simulink model "sixth"  (R2021b)
settings: Solver=ode45  StartTime=0.0  StopTime=50  RelTol=1e-3
libraries: simulink x3
settings Model: Creator=minna  LastModifiedBy=minna

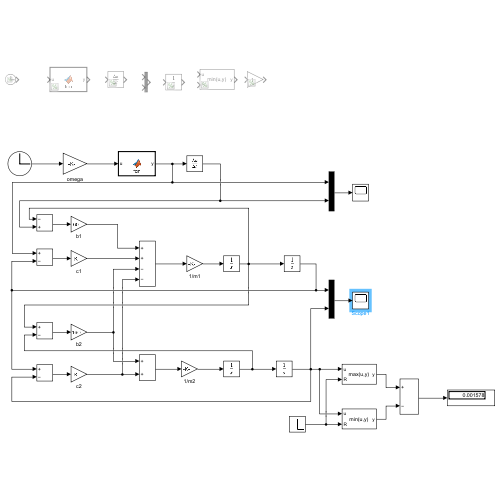
[thumbnail: Simulink's stored preview of the top-level diagram]
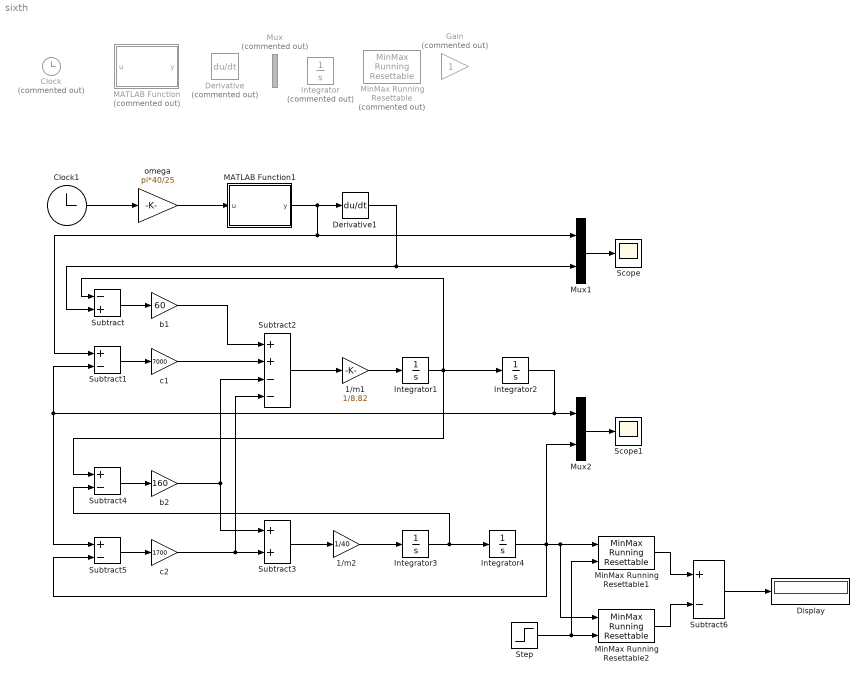
== system sixth ==
  1/m1 : Gain  Gain=1/8.82
  1/m2 : Gain  Gain=1/40
  Clock : Clock  Commented=on
  Clock1 : Clock
  Derivative : Derivative  Commented=on
  Derivative1 : Derivative
  Display : Display
  Gain : Gain  Commented=on
  Integrator : Integrator  Commented=on
  Integrator{1..4} (4 alike) : Integrator
  MATLAB Function : MATLAB Function  Commented=on  TreatAsAtomicUnit=on
  MATLAB Function1 : MATLAB Function  TreatAsAtomicUnit=on
  MinMax Running Resettable : simulink/Math Operations/MinMax Running Resettable  Commented=on  Function=min  vinit=0.0
  MinMax Running Resettable1 : simulink/Math Operations/MinMax Running Resettable  Function=max  vinit=0.0
  MinMax Running Resettable2 : simulink/Math Operations/MinMax Running Resettable  Function=min  vinit=10
  Mux : Mux  Commented=on  Inputs=2
  Mux1 : Mux  Inputs=2
  Mux2 : Mux  Inputs=2
  Scope : Scope
  Scope1 : Scope
  Step : Step  Time=10  Before=1  After=0  SampleTime=0
  Subtract : Sum  Inputs=-+
  Subtract{1,4..6} (4 alike) : Sum  Inputs=+-
  Subtract2 : Sum  Inputs=++--
  Subtract3 : Sum
  b1 : Gain  Gain=60
  b2 : Gain  Gain=160
  c1 : Gain  Gain=7000
  c2 : Gain  Gain=1700
  omega : Gain  Gain=pi*40/25
  wires:
  Clock1/1 -> omega/1
  omega/1 -> MATLAB Function1/1(u)
  MATLAB Function1/1(y) -> Subtract1/1, Mux1/1, Derivative1/1
  Derivative1/1 -> Mux1/2, Subtract/2
  Subtract/1 -> b1/1
  Subtract1/1 -> c1/1
  c1/1 -> Subtract2/2
  b1/1 -> Subtract2/1
  Subtract2/1 -> 1/m1/1
  1/m1/1 -> Integrator1/1
  Integrator1/1 -> Subtract4/1, Integrator2/1, Subtract/1
  Integrator2/1 -> Mux2/1, Subtract5/1, Subtract1/2
  Mux1/1 -> Scope/1
  Mux2/1 -> Scope1/1
  b2/1 -> Subtract3/1, Subtract2/3
  Subtract4/1 -> b2/1
  Subtract5/1 -> c2/1
  c2/1 -> Subtract2/4, Subtract3/2
  Subtract3/1 -> 1/m2/1
  1/m2/1 -> Integrator3/1
  Integrator3/1 -> Integrator4/1, Subtract4/2
  Integrator4/1 -> Mux2/2, MinMax Running Resettable2/1, MinMax Running Resettable1/1, Subtract5/2
  Step/1 -> MinMax Running Resettable1/2, MinMax Running Resettable2/2
  MinMax Running Resettable1/1 -> Subtract6/1
  MinMax Running Resettable2/1 -> Subtract6/2
  Subtract6/1 -> Display/1

== matlab function sixth/MATLAB Function ==
  data: u input; y output
function y = fcn(u)

y = abs(0.005*sin(u)+0.002*sin(3*u));

== matlab function sixth/MATLAB Function1 ==
  data: u input; y output
function y = fcn(u)

y = abs(0.005*sin(u)+0.002*sin(3*u));
